simulink library "sm_rollerV_lib_underc_idlerArm_i2u0l3"  (R2026a)
settings: Solver=VariableStepAuto
undefined symbols (not defined in the file): Fixed, P1, P2, P3, P4, P5, Right, Trac, X, Y, Z
libraries: sm_rollerV_lib_underc_elem x11, sm_lib x11, nesl_utility x7, sm_trackV_lib_belt_underc_elem x4, fl_lib x2, sm_trackV_lib_frame_idlerArm_i2u0l3 x1
(part 2 of 2)

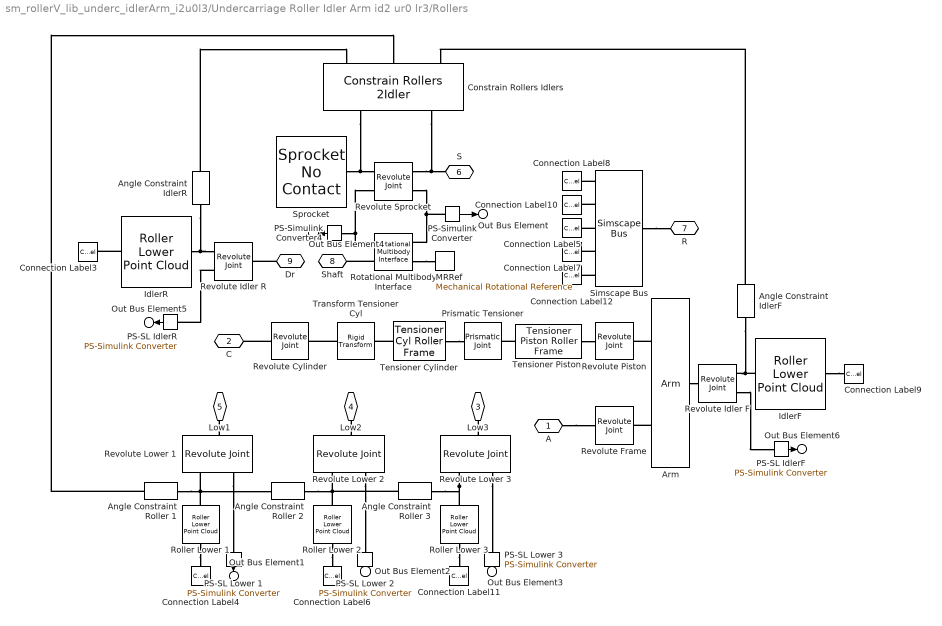
== system sm_rollerV_lib_underc_idlerArm_i2u0l3/Undercarriage Roller Idler Arm id2 ur0 lr3/Rollers ==
  Angle Constraint IdlerF : sm_rollerV_lib_underc_elem/Angle Constraint  SystemSampleTime=-1  VariantActivationTime=update diagram  EmptyChoice=off  PassThrough=off  PassThroughVariantControl=(default)  EmptyChoiceVariantControl=(default)  AllowFlexibleInterface=on  Latency=0  AutoFrameSizeCalculation=off
  Angle Constraint IdlerR : sm_rollerV_lib_underc_elem/Angle Constraint  SystemSampleTime=-1  VariantActivationTime=update diagram  EmptyChoice=off  PassThrough=off  PassThroughVariantControl=(default)  EmptyChoiceVariantControl=(default)  AllowFlexibleInterface=on  Latency=0  AutoFrameSizeCalculation=off
  Angle Constraint Roller 1 : sm_rollerV_lib_underc_elem/Angle Constraint  SystemSampleTime=-1  VariantActivationTime=update diagram  EmptyChoice=off  PassThrough=off  PassThroughVariantControl=(default)  EmptyChoiceVariantControl=(default)  AllowFlexibleInterface=on  Latency=0  AutoFrameSizeCalculation=off
  Angle Constraint Roller 2 : sm_rollerV_lib_underc_elem/Angle Constraint  SystemSampleTime=-1  VariantActivationTime=update diagram  EmptyChoice=off  PassThrough=off  PassThroughVariantControl=(default)  EmptyChoiceVariantControl=(default)  AllowFlexibleInterface=on  Latency=0  AutoFrameSizeCalculation=off
  Angle Constraint Roller 3 : sm_rollerV_lib_underc_elem/Angle Constraint  SystemSampleTime=-1  VariantActivationTime=update diagram  EmptyChoice=off  PassThrough=off  PassThroughVariantControl=(default)  EmptyChoiceVariantControl=(default)  AllowFlexibleInterface=on  Latency=0  AutoFrameSizeCalculation=off
  Arm : sm_trackV_lib_belt_underc_elem/Arm  arm_idlerc=arm_idlerc  arm_tens_x=arm_tens_x  arm_tens_y=arm_tens_y  arm_wid=arm_wid  arm_thk=arm_thk  arm_rho=arm_rho  arm_clr=arm_clr  arm_opc=arm_opc
  Connection Label10 : ConnectionLabel  Label=A
  Connection Label11 : ConnectionLabel  Label=L3
  Connection Label12 : ConnectionLabel  Label=L3
  Connection Label3 : ConnectionLabel  Label=X
  Connection Label4 : ConnectionLabel  Label=L1
  Connection Label5 : ConnectionLabel  Label=L1
  Connection Label6 : ConnectionLabel  Label=L2
  Connection Label7 : ConnectionLabel  Label=L2
  Connection Label8 : ConnectionLabel  Label=X
  Connection Label9 : ConnectionLabel  Label=A
  Constrain Rollers Idlers : sm_rollerV_lib_underc_elem/Constrain Rollers 2Idler  sprk_rolling_rad=sprk_rolling_rad  roller_lower_rolling_rad=roller_lower_rolling_rad  idlerF_rolling_rad=idlerF_rolling_rad  idlerR_rolling_rad=idlerR_rolling_rad
  IdlerF : sm_rollerV_lib_underc_elem/Roller Lower Point Cloud  roller_lower_rad=idlerF_rad  roller_lower_len=idlerF_total_len  roller_lower_rho=idlerF_avg_rho  roller_lower_clr=idlerF_clr  roller_lower_opc=idlerF_opc  roller_lower_contgeo_ptcld=idlerF_contgeo_ptcld  roller_lower_contgeo_rad=idlerF_contgeo_rad  roller_lower_contgeo_clr=idlerF_contgeo_clr  roller_lower_contgeo_opc=idlerF_contgeo_opc  cyl_rad=idlerF_rolling_rad  cyl_len=cyl_len  cyl_clr=idlerF_rollvervis_clr  cyl_opc=idlerF_rollervis_opc  accMn=accMn  accMx=accMx  acc_clr=acc_clr  acc_opc=acc_opc  lext=lext
      settings: LibrarySourceBlock=sm_chain_drive_lib/Pulley_Bot
  IdlerR : sm_rollerV_lib_underc_elem/Roller Lower Point Cloud  roller_lower_rad=idlerR_rad  roller_lower_len=idlerR_total_len  roller_lower_rho=idlerR_avg_rho  roller_lower_clr=idlerR_clr  roller_lower_opc=idlerR_opc  roller_lower_contgeo_ptcld=idlerR_contgeo_ptcld  roller_lower_contgeo_rad=idlerR_contgeo_rad  roller_lower_contgeo_clr=idlerR_contgeo_clr  roller_lower_contgeo_opc=idlerR_contgeo_opc  cyl_rad=idlerR_rolling_rad  cyl_len=cyl_len  cyl_clr=idlerR_rollvervis_clr  cyl_opc=idlerR_rollervis_opc  accMn=accMn  accMx=accMx  acc_clr=acc_clr  acc_opc=acc_opc  lext=lext
      settings: LibrarySourceBlock=sm_chain_drive_lib/Pulley_Bot
  MRRef : fl_lib/Mechanical/Rotational Elements/Mechanical Rotational Reference
  PS-SL IdlerF : nesl_utility/PS-Simulink Converter  PhysicalDomain=network_engine_domain  SubClassName=ps_output  LeftPortType=input  RightPortType=output  PseudoPeriodic=off  Frequencies=[]  VectorFormat=inherit  Unit=inherit  AffineConversion=off
  PS-SL IdlerR : nesl_utility/PS-Simulink Converter  PhysicalDomain=network_engine_domain  SubClassName=ps_output  LeftPortType=input  RightPortType=output  PseudoPeriodic=off  Frequencies=[]  VectorFormat=inherit  Unit=inherit  AffineConversion=off
  PS-SL Lower 1 : nesl_utility/PS-Simulink Converter  PhysicalDomain=network_engine_domain  SubClassName=ps_output  LeftPortType=input  RightPortType=output  PseudoPeriodic=off  Frequencies=[]  VectorFormat=inherit  Unit=inherit  AffineConversion=off
  PS-SL Lower 2 : nesl_utility/PS-Simulink Converter  PhysicalDomain=network_engine_domain  SubClassName=ps_output  LeftPortType=input  RightPortType=output  PseudoPeriodic=off  Frequencies=[]  VectorFormat=inherit  Unit=inherit  AffineConversion=off
  PS-SL Lower 3 : nesl_utility/PS-Simulink Converter  PhysicalDomain=network_engine_domain  SubClassName=ps_output  LeftPortType=input  RightPortType=output  PseudoPeriodic=off  Frequencies=[]  VectorFormat=inherit  Unit=inherit  AffineConversion=off
  PS-Simulink Converter : nesl_utility/PS-Simulink Converter  PhysicalDomain=network_engine_domain  SubClassName=ps_output  LeftPortType=input  RightPortType=output  PseudoPeriodic=off  Frequencies=[]  VectorFormat=inherit  Unit=inherit  AffineConversion=off
  PS-Simulink Converter4 : nesl_utility/PS-Simulink Converter  PhysicalDomain=network_engine_domain  SubClassName=ps_output  LeftPortType=input  RightPortType=output  PseudoPeriodic=off  Frequencies=[]  VectorFormat=inherit  Unit=inherit  AffineConversion=off
  Prismatic Tensioner : sm_lib/Joints/Prismatic Joint  JointMode=Normal  CompositeWrenchDir=FollowerOnBase  CompositeWrenchFrame=BaseFrame  SenseConstraintForce=off  SenseConstraintTorque=off  SenseTotalForce=off  SenseTotalTorque=off  PositionTargetSpecify=on  PositionTargetPriority=High  PositionTargetValue=tensioner_x0  PositionTargetValueUnits=m  VelocityTargetSpecify=off  VelocityTargetPriority=High  VelocityTargetValue=0  VelocityTargetValueUnits=m/s  EquilibriumPosition=tensioner_eqpos  EquilibriumPositionUnits=m  SpringStiffness=tensioner_k  SpringStiffnessUnits=N/m  DampingCoefficient=tensioner_b  DampingCoefficientUnits=N/(m/s)  LowerLimitSpecify=off  LowerLimitBound=-1  LowerLimitBoundUnits=m  LowerLimitStiffness=1e6  LowerLimitStiffnessUnits=N/m  LowerLimitDamping=1e3  LowerLimitDampingUnits=N/(m/s)  LowerLimitTransitionRegionWidth=1e-4  LowerLimitTransitionRegionWidthUnits=m  UpperLimitSpecify=off  UpperLimitBound=1  UpperLimitBoundUnits=m  UpperLimitStiffness=1e6  UpperLimitStiffnessUnits=N/m  UpperLimitDamping=1e3  UpperLimitDampingUnits=N/(m/s)  UpperLimitTransitionRegionWidth=1e-4  UpperLimitTransitionRegionWidthUnits=m  TorqueActuationMode=NoTorque  MotionActuationMode=ComputedMotion  SensePosition=off  SenseVelocity=off  SenseAcceleration=off  SenseTorqueForce=off  SenseLowerLimitTorqueForce=off  SenseUpperLimitTorqueForce=off
  Revolute Cylinder : sm_lib/Joints/Revolute Joint  JointMode=Normal  CompositeWrenchDir=FollowerOnBase  CompositeWrenchFrame=BaseFrame  SenseConstraintForce=off  SenseConstraintTorque=off  SenseTotalForce=off  SenseTotalTorque=off  PositionTargetSpecify=on  PositionTargetPriority=Low  PositionTargetValue=0  PositionTargetValueUnits=deg  VelocityTargetSpecify=off  VelocityTargetPriority=High  VelocityTargetValue=0  VelocityTargetValueUnits=deg/s  EquilibriumPosition=0  EquilibriumPositionUnits=deg  SpringStiffness=0  SpringStiffnessUnits=N*m/deg  DampingCoefficient=0  DampingCoefficientUnits=N*m/(deg/s)  LowerLimitSpecify=off  LowerLimitBound=-90  LowerLimitBoundUnits=deg  LowerLimitStiffness=1e4  LowerLimitStiffnessUnits=N*m/deg  LowerLimitDamping=10  LowerLimitDampingUnits=N*m/(deg/s)  LowerLimitTransitionRegionWidth=0.1  LowerLimitTransitionRegionWidthUnits=deg  UpperLimitSpecify=off  UpperLimitBound=90  UpperLimitBoundUnits=deg  UpperLimitStiffness=1e4  UpperLimitStiffnessUnits=N*m/deg  UpperLimitDamping=10  UpperLimitDampingUnits=N*m/(deg/s)  UpperLimitTransitionRegionWidth=0.1  UpperLimitTransitionRegionWidthUnits=deg  TorqueActuationMode=NoTorque  MotionActuationMode=ComputedMotion  SensePosition=off  SenseVelocity=off  SenseAcceleration=off  SenseTorqueForce=off  SenseLowerLimitTorqueForce=off  SenseUpperLimitTorqueForce=off
  Revolute Frame : sm_lib/Joints/Revolute Joint  JointMode=Normal  CompositeWrenchDir=FollowerOnBase  CompositeWrenchFrame=BaseFrame  SenseConstraintForce=off  SenseConstraintTorque=off  SenseTotalForce=off  SenseTotalTorque=off  PositionTargetSpecify=off  PositionTargetPriority=Low  PositionTargetValue=0  PositionTargetValueUnits=deg  VelocityTargetSpecify=off  VelocityTargetPriority=High  VelocityTargetValue=0  VelocityTargetValueUnits=deg/s  EquilibriumPosition=0  EquilibriumPositionUnits=rad  SpringStiffness=0  SpringStiffnessUnits=N*m/rad  DampingCoefficient=0  DampingCoefficientUnits=N*m/(rad/s)  LowerLimitSpecify=off  LowerLimitBound=-90  LowerLimitBoundUnits=deg  LowerLimitStiffness=1e4  LowerLimitStiffnessUnits=N*m/deg  LowerLimitDamping=10  LowerLimitDampingUnits=N*m/(deg/s)  LowerLimitTransitionRegionWidth=0.1  LowerLimitTransitionRegionWidthUnits=deg  UpperLimitSpecify=off  UpperLimitBound=90  UpperLimitBoundUnits=deg  UpperLimitStiffness=1e4  UpperLimitStiffnessUnits=N*m/deg  UpperLimitDamping=10  UpperLimitDampingUnits=N*m/(deg/s)  UpperLimitTransitionRegionWidth=0.1  UpperLimitTransitionRegionWidthUnits=deg  TorqueActuationMode=NoTorque  MotionActuationMode=ComputedMotion  SensePosition=off  SenseVelocity=off  SenseAcceleration=off  SenseTorqueForce=off  SenseLowerLimitTorqueForce=off  SenseUpperLimitTorqueForce=off
  Revolute Idler F : sm_lib/Joints/Revolute Joint  JointMode=Normal  CompositeWrenchDir=FollowerOnBase  CompositeWrenchFrame=BaseFrame  SenseConstraintForce=off  SenseConstraintTorque=off  SenseTotalForce=off  SenseTotalTorque=off  PositionTargetSpecify=off  PositionTargetPriority=Low  PositionTargetValue=0  PositionTargetValueUnits=deg  VelocityTargetSpecify=off  VelocityTargetPriority=High  VelocityTargetValue=0  VelocityTargetValueUnits=deg/s  EquilibriumPosition=0  EquilibriumPositionUnits=rad  SpringStiffness=0  SpringStiffnessUnits=N*m/rad  DampingCoefficient=0  DampingCoefficientUnits=N*m/(rad/s)  LowerLimitSpecify=off  LowerLimitBound=-90  LowerLimitBoundUnits=deg  LowerLimitStiffness=1e4  LowerLimitStiffnessUnits=N*m/deg  LowerLimitDamping=10  LowerLimitDampingUnits=N*m/(deg/s)  LowerLimitTransitionRegionWidth=0.1  LowerLimitTransitionRegionWidthUnits=deg  UpperLimitSpecify=off  UpperLimitBound=90  UpperLimitBoundUnits=deg  UpperLimitStiffness=1e4  UpperLimitStiffnessUnits=N*m/deg  UpperLimitDamping=10  UpperLimitDampingUnits=N*m/(deg/s)  UpperLimitTransitionRegionWidth=0.1  UpperLimitTransitionRegionWidthUnits=deg  TorqueActuationMode=NoTorque  MotionActuationMode=ComputedMotion  SensePosition=off  SenseVelocity=off  SenseAcceleration=off  SenseTorqueForce=on  SenseLowerLimitTorqueForce=off  SenseUpperLimitTorqueForce=off
  Revolute Idler R : sm_lib/Joints/Revolute Joint  JointMode=Normal  CompositeWrenchDir=FollowerOnBase  CompositeWrenchFrame=BaseFrame  SenseConstraintForce=off  SenseConstraintTorque=off  SenseTotalForce=off  SenseTotalTorque=off  PositionTargetSpecify=off  PositionTargetPriority=Low  PositionTargetValue=0  PositionTargetValueUnits=deg  VelocityTargetSpecify=off  VelocityTargetPriority=High  VelocityTargetValue=0  VelocityTargetValueUnits=deg/s  EquilibriumPosition=0  EquilibriumPositionUnits=rad  SpringStiffness=0  SpringStiffnessUnits=N*m/rad  DampingCoefficient=0  DampingCoefficientUnits=N*m/(rad/s)  LowerLimitSpecify=off  LowerLimitBound=-90  LowerLimitBoundUnits=deg  LowerLimitStiffness=1e4  LowerLimitStiffnessUnits=N*m/deg  LowerLimitDamping=10  LowerLimitDampingUnits=N*m/(deg/s)  LowerLimitTransitionRegionWidth=0.1  LowerLimitTransitionRegionWidthUnits=deg  UpperLimitSpecify=off  UpperLimitBound=90  UpperLimitBoundUnits=deg  UpperLimitStiffness=1e4  UpperLimitStiffnessUnits=N*m/deg  UpperLimitDamping=10  UpperLimitDampingUnits=N*m/(deg/s)  UpperLimitTransitionRegionWidth=0.1  UpperLimitTransitionRegionWidthUnits=deg  TorqueActuationMode=NoTorque  MotionActuationMode=ComputedMotion  SensePosition=off  SenseVelocity=off  SenseAcceleration=off  SenseTorqueForce=on  SenseLowerLimitTorqueForce=off  SenseUpperLimitTorqueForce=off
  Revolute Lower 1 : sm_lib/Joints/Revolute Joint  JointMode=Normal  CompositeWrenchDir=FollowerOnBase  CompositeWrenchFrame=BaseFrame  SenseConstraintForce=off  SenseConstraintTorque=off  SenseTotalForce=off  SenseTotalTorque=off  PositionTargetSpecify=off  PositionTargetPriority=Low  PositionTargetValue=0  PositionTargetValueUnits=deg  VelocityTargetSpecify=off  VelocityTargetPriority=High  VelocityTargetValue=0  VelocityTargetValueUnits=deg/s  EquilibriumPosition=0  EquilibriumPositionUnits=rad  SpringStiffness=0  SpringStiffnessUnits=N*m/rad  DampingCoefficient=0  DampingCoefficientUnits=N*m/(rad/s)  LowerLimitSpecify=off  LowerLimitBound=-90  LowerLimitBoundUnits=deg  LowerLimitStiffness=1e4  LowerLimitStiffnessUnits=N*m/deg  LowerLimitDamping=10  LowerLimitDampingUnits=N*m/(deg/s)  LowerLimitTransitionRegionWidth=0.1  LowerLimitTransitionRegionWidthUnits=deg  UpperLimitSpecify=off  UpperLimitBound=90  UpperLimitBoundUnits=deg  UpperLimitStiffness=1e4  UpperLimitStiffnessUnits=N*m/deg  UpperLimitDamping=10  UpperLimitDampingUnits=N*m/(deg/s)  UpperLimitTransitionRegionWidth=0.1  UpperLimitTransitionRegionWidthUnits=deg  TorqueActuationMode=NoTorque  MotionActuationMode=ComputedMotion  SensePosition=off  SenseVelocity=off  SenseAcceleration=off  SenseTorqueForce=on  SenseLowerLimitTorqueForce=off  SenseUpperLimitTorqueForce=off
  Revolute Lower 2 : sm_lib/Joints/Revolute Joint  JointMode=Normal  CompositeWrenchDir=FollowerOnBase  CompositeWrenchFrame=BaseFrame  SenseConstraintForce=off  SenseConstraintTorque=off  SenseTotalForce=off  SenseTotalTorque=off  PositionTargetSpecify=off  PositionTargetPriority=Low  PositionTargetValue=0  PositionTargetValueUnits=deg  VelocityTargetSpecify=off  VelocityTargetPriority=High  VelocityTargetValue=0  VelocityTargetValueUnits=deg/s  EquilibriumPosition=0  EquilibriumPositionUnits=rad  SpringStiffness=0  SpringStiffnessUnits=N*m/rad  DampingCoefficient=0  DampingCoefficientUnits=N*m/(rad/s)  LowerLimitSpecify=off  LowerLimitBound=-90  LowerLimitBoundUnits=deg  LowerLimitStiffness=1e4  LowerLimitStiffnessUnits=N*m/deg  LowerLimitDamping=10  LowerLimitDampingUnits=N*m/(deg/s)  LowerLimitTransitionRegionWidth=0.1  LowerLimitTransitionRegionWidthUnits=deg  UpperLimitSpecify=off  UpperLimitBound=90  UpperLimitBoundUnits=deg  UpperLimitStiffness=1e4  UpperLimitStiffnessUnits=N*m/deg  UpperLimitDamping=10  UpperLimitDampingUnits=N*m/(deg/s)  UpperLimitTransitionRegionWidth=0.1  UpperLimitTransitionRegionWidthUnits=deg  TorqueActuationMode=NoTorque  MotionActuationMode=ComputedMotion  SensePosition=off  SenseVelocity=off  SenseAcceleration=off  SenseTorqueForce=on  SenseLowerLimitTorqueForce=off  SenseUpperLimitTorqueForce=off
  Revolute Lower 3 : sm_lib/Joints/Revolute Joint  JointMode=Normal  CompositeWrenchDir=FollowerOnBase  CompositeWrenchFrame=BaseFrame  SenseConstraintForce=off  SenseConstraintTorque=off  SenseTotalForce=off  SenseTotalTorque=off  PositionTargetSpecify=off  PositionTargetPriority=Low  PositionTargetValue=0  PositionTargetValueUnits=deg  VelocityTargetSpecify=off  VelocityTargetPriority=High  VelocityTargetValue=0  VelocityTargetValueUnits=deg/s  EquilibriumPosition=0  EquilibriumPositionUnits=rad  SpringStiffness=0  SpringStiffnessUnits=N*m/rad  DampingCoefficient=0  DampingCoefficientUnits=N*m/(rad/s)  LowerLimitSpecify=off  LowerLimitBound=-90  LowerLimitBoundUnits=deg  LowerLimitStiffness=1e4  LowerLimitStiffnessUnits=N*m/deg  LowerLimitDamping=10  LowerLimitDampingUnits=N*m/(deg/s)  LowerLimitTransitionRegionWidth=0.1  LowerLimitTransitionRegionWidthUnits=deg  UpperLimitSpecify=off  UpperLimitBound=90  UpperLimitBoundUnits=deg  UpperLimitStiffness=1e4  UpperLimitStiffnessUnits=N*m/deg  UpperLimitDamping=10  UpperLimitDampingUnits=N*m/(deg/s)  UpperLimitTransitionRegionWidth=0.1  UpperLimitTransitionRegionWidthUnits=deg  TorqueActuationMode=NoTorque  MotionActuationMode=ComputedMotion  SensePosition=off  SenseVelocity=off  SenseAcceleration=off  SenseTorqueForce=on  SenseLowerLimitTorqueForce=off  SenseUpperLimitTorqueForce=off
  Revolute Piston : sm_lib/Joints/Revolute Joint  JointMode=Normal  CompositeWrenchDir=FollowerOnBase  CompositeWrenchFrame=BaseFrame  SenseConstraintForce=off  SenseConstraintTorque=off  SenseTotalForce=off  SenseTotalTorque=off  PositionTargetSpecify=off  PositionTargetPriority=Low  PositionTargetValue=0  PositionTargetValueUnits=deg  VelocityTargetSpecify=off  VelocityTargetPriority=High  VelocityTargetValue=0  VelocityTargetValueUnits=deg/s  EquilibriumPosition=0  EquilibriumPositionUnits=rad  SpringStiffness=0  SpringStiffnessUnits=N*m/rad  DampingCoefficient=0  DampingCoefficientUnits=N*m/(rad/s)  LowerLimitSpecify=off  LowerLimitBound=-90  LowerLimitBoundUnits=deg  LowerLimitStiffness=1e4  LowerLimitStiffnessUnits=N*m/deg  LowerLimitDamping=10  LowerLimitDampingUnits=N*m/(deg/s)  LowerLimitTransitionRegionWidth=0.1  LowerLimitTransitionRegionWidthUnits=deg  UpperLimitSpecify=off  UpperLimitBound=90  UpperLimitBoundUnits=deg  UpperLimitStiffness=1e4  UpperLimitStiffnessUnits=N*m/deg  UpperLimitDamping=10  UpperLimitDampingUnits=N*m/(deg/s)  UpperLimitTransitionRegionWidth=0.1  UpperLimitTransitionRegionWidthUnits=deg  TorqueActuationMode=NoTorque  MotionActuationMode=ComputedMotion  SensePosition=off  SenseVelocity=off  SenseAcceleration=off  SenseTorqueForce=off  SenseLowerLimitTorqueForce=off  SenseUpperLimitTorqueForce=off
  Revolute Sprocket : sm_lib/Joints/Revolute Joint  JointMode=Normal  CompositeWrenchDir=FollowerOnBase  CompositeWrenchFrame=BaseFrame  SenseConstraintForce=off  SenseConstraintTorque=off  SenseTotalForce=off  SenseTotalTorque=off  PositionTargetSpecify=off  PositionTargetPriority=Low  PositionTargetValue=0  PositionTargetValueUnits=deg  VelocityTargetSpecify=off  VelocityTargetPriority=High  VelocityTargetValue=0  VelocityTargetValueUnits=deg/s  EquilibriumPosition=0  EquilibriumPositionUnits=rad  SpringStiffness=0  SpringStiffnessUnits=N*m/rad  DampingCoefficient=0  DampingCoefficientUnits=N*m/(rad/s)  LowerLimitSpecify=off  LowerLimitBound=-90  LowerLimitBoundUnits=deg  LowerLimitStiffness=1e4  LowerLimitStiffnessUnits=N*m/deg  LowerLimitDamping=10  LowerLimitDampingUnits=N*m/(deg/s)  LowerLimitTransitionRegionWidth=0.1  LowerLimitTransitionRegionWidthUnits=deg  UpperLimitSpecify=off  UpperLimitBound=90  UpperLimitBoundUnits=deg  UpperLimitStiffness=1e4  UpperLimitStiffnessUnits=N*m/deg  UpperLimitDamping=10  UpperLimitDampingUnits=N*m/(deg/s)  UpperLimitTransitionRegionWidth=0.1  UpperLimitTransitionRegionWidthUnits=deg  TorqueActuationMode=InputTorque  MotionActuationMode=ComputedMotion  SensePosition=off  SenseVelocity=on  SenseAcceleration=off  SenseTorqueForce=off  SenseLowerLimitTorqueForce=off  SenseUpperLimitTorqueForce=off
  Roller Lower 1 : sm_rollerV_lib_underc_elem/Roller Lower Point Cloud  roller_lower_rad=roller_lower_rad  roller_lower_len=roller_lower_len  roller_lower_rho=roller_lower_rho  roller_lower_clr=roller_lower_clr  roller_lower_opc=roller_lower_opc  roller_lower_contgeo_ptcld=roller_lower_contgeo_ptcld  roller_lower_contgeo_rad=roller_lower_contgeo_rad  roller_lower_contgeo_clr=roller_lower_contgeo_clr  roller_lower_contgeo_opc=roller_lower_contgeo_opc  cyl_rad=roller_lower_rolling_rad  cyl_len=cyl_len  cyl_clr=roller_lower_cyl_clr  cyl_opc=roller_lower_cyl_opc  accMn=accMn  accMx=accMx  acc_clr=acc_clr  acc_opc=acc_opc  lext=lext
      settings: LibrarySourceBlock=sm_chain_drive_lib/Pulley_Bot
  Roller Lower 2 : sm_rollerV_lib_underc_elem/Roller Lower Point Cloud  roller_lower_rad=roller_lower_rad  roller_lower_len=roller_lower_len  roller_lower_rho=roller_lower_rho  roller_lower_clr=roller_lower_clr  roller_lower_opc=roller_lower_opc  roller_lower_contgeo_ptcld=roller_lower_contgeo_ptcld  roller_lower_contgeo_rad=roller_lower_contgeo_rad  roller_lower_contgeo_clr=roller_lower_contgeo_clr  roller_lower_contgeo_opc=roller_lower_contgeo_opc  cyl_rad=roller_lower_rolling_rad  cyl_len=cyl_len  cyl_clr=roller_lower_cyl_clr  cyl_opc=roller_lower_cyl_opc  accMn=accMn  accMx=accMx  acc_clr=acc_clr  acc_opc=acc_opc  lext=lext
      settings: LibrarySourceBlock=sm_chain_drive_lib/Pulley_Bot
  Roller Lower 3 : sm_rollerV_lib_underc_elem/Roller Lower Point Cloud  roller_lower_rad=roller_lower_rad  roller_lower_len=roller_lower_len  roller_lower_rho=roller_lower_rho  roller_lower_clr=roller_lower_clr  roller_lower_opc=roller_lower_opc  roller_lower_contgeo_ptcld=roller_lower_contgeo_ptcld  roller_lower_contgeo_rad=roller_lower_contgeo_rad  roller_lower_contgeo_clr=roller_lower_contgeo_clr  roller_lower_contgeo_opc=roller_lower_contgeo_opc  cyl_rad=roller_lower_rolling_rad  cyl_len=cyl_len  cyl_clr=roller_lower_cyl_clr  cyl_opc=roller_lower_cyl_opc  accMn=accMn  accMx=accMx  acc_clr=acc_clr  acc_opc=acc_opc  lext=lext
      settings: LibrarySourceBlock=sm_chain_drive_lib/Pulley_Bot
  Rotational Multibody Interface : fl_lib/Mechanical/Multibody Interfaces/Rotational Multibody Interface
  Simscape Bus : SimscapeBus  HierarchyStrings=P1;P2;P3;P4;P5
  Sprocket : sm_trackV_lib_belt_underc_elem/Sprocket No Contact  sprk_wid_roll=sprk_wid_roll  sprk_rad_roll=sprk_rad_roll  sprk_opc=sprk_opc  sprk_clr=sprk_clr  sprk_rad_pitch=sprk_rad_pitch  sprk_spoke_rad=sprk_spoke_rad  sprk_spoke_len=sprk_spoke_len  sprk_spoke_num=sprk_spoke_num  sprk_spoke_clr=sprk_clr  sprk_spoke_opc=sprk_opc  rim_spoke_xc=sprk_rim_spoke_xc  rim_thk=sprk_rim_thk  rim_ir=sprk_rim_ir
  Tensioner Cylinder : sm_trackV_lib_belt_underc_elem/Tensioner Cyl Roller Frame  cyl_rad=tensioner_cyl_rad  cyl_len=tensioner_cyl_len  cyl_rho=tensioner_cyl_rho  cyl_clr=tensioner_cyl_clr  cyl_opc=tensioner_cyl_opc
  Tensioner Piston : sm_trackV_lib_belt_underc_elem/Tensioner Piston Roller Frame  pist_rad=tensioner_pist_rad  pist_len=pist_len  pist_rho=tensioner_pist_rho  pist_clr=tensioner_pist_clr  pist_opc=tensioner_pist_opc  br_height=tensioner_br_height  br_length=brk_len  br_width=tensioner_br_width  br_rho=tensioner_br_rho  br_thk=brk_thk  br_clr=tensioner_br_clr  br_opc=tensioner_br_opc
  Transform Tensioner Cyl : sm_lib/Frames and Transforms/Rigid Transform  RotationMethod=AlignedAxes  FollAlignAxisA=+Z  BaseAlignAxisA=+X  FollAlignAxisB=+X  BaseAlignAxisB=+Y  RotationStandardAxis=+Y  RotationAngle=90  RotationAngleUnits=deg  RotationArbitraryAxis=[0 0 1]  RotationSequenceAxes=FollowerAxes  RotationSequence=XYX  RotationSequenceAngles=[0 0 0]  RotationSequenceAnglesUnits=deg  RotationMatrix=[1 0 0; 0 1 0; 0 0 1]  Quaternion=[1 0 0 0]  TranslationMethod=None  TranslationCartesianOffset=[0 0 0]  TranslationCartesianOffsetUnits=m  TranslationStandardAxis=+Z  TranslationStandardOffset=0  TranslationStandardOffsetUnits=m  TranslationROffset=0  TranslationROffsetUnits=m  TranslationThetaOffset=0  TranslationThetaOffsetUnits=deg  TranslationZOffset=0  TranslationZOffsetUnits=m
  A : PMIOPort  Side=Left
  C : PMIOPort  Port=2  Side=Left
  Low3 : PMIOPort  Port=3  Side=Left
  Low2 : PMIOPort  Port=4  Side=Left
  Low1 : PMIOPort  Port=5  Side=Left
  S : PMIOPort  Port=6  Side=Left
  R : PMIOPort  Port=7  Side=Right
  Shaft : PMIOPort  Port=8  Side=Right
  Dr : PMIOPort  Port=9  Side=Left
  Out Bus Element : Outport  PortName=m  Element=tSprk
  Out Bus Element1 : Outport  PortName=m  Element=RL1
  Out Bus Element2 : Outport  PortName=m  Element=RL2
  Out Bus Element3 : Outport  PortName=m  Element=RL3
  Out Bus Element4 : Outport  PortName=m  Element=wSprk
  Out Bus Element5 : Outport  PortName=m  Element=XIdlerR
  Out Bus Element6 : Outport  PortName=m  Element=XIdlerF
  wires:
  PS-Simulink Converter/1 -> Out Bus Element/1
  PS-SL Lower 1/1 -> Out Bus Element1/1
  PS-SL Lower 2/1 -> Out Bus Element2/1
  PS-SL Lower 3/1 -> Out Bus Element3/1
  PS-Simulink Converter4/1 -> Out Bus Element4/1
  PS-SL IdlerR/1 -> Out Bus Element5/1
  PS-SL IdlerF/1 -> Out Bus Element6/1
  connections:
  A/RConn1 -- Revolute Frame/LConn1
  Arm/LConn2 -- Revolute Frame/RConn1
  Tensioner Piston/RConn1 -- Revolute Piston/LConn1
  Arm/LConn1 -- Revolute Piston/RConn1
  Arm/RConn1 -- Revolute Idler F/LConn1
  IdlerF/RConn1 -- Connection Label9/LConn1
  Roller Lower 2/RConn1 -- Connection Label6/LConn1
  Revolute Sprocket/LConn1 -- Constrain Rollers Idlers/LConn2 -- S/RConn1
  Simscape Bus/RConn1 -- R/RConn1
  IdlerF/LConn1 -- Angle Constraint IdlerF/RConn1 -- Revolute Idler F/RConn1
  Revolute Sprocket/RConn1 -- Constrain Rollers Idlers/LConn1 -- Sprocket/RConn1
  Tensioner Cylinder/RConn1 -- Prismatic Tensioner/LConn1
  Revolute Lower 2/LConn1 -- Low2/RConn1
  Roller Lower 1/RConn1 -- Connection Label4/LConn1
  Revolute Lower 1/LConn1 -- Low1/RConn1
  Simscape Bus/LConn1 -- Connection Label8/LConn1
  Tensioner Cylinder/LConn1 -- Transform Tensioner Cyl/RConn1
  Tensioner Piston/LConn1 -- Prismatic Tensioner/RConn1
  Angle Constraint Roller 2/RConn1 -- Roller Lower 2/LConn1 -- Angle Constraint Roller 3/LConn1 -- Revolute Lower 2/RConn1
  Angle Constraint Roller 1/RConn1 -- Roller Lower 1/LConn1 -- Angle Constraint Roller 2/LConn1 -- Revolute Lower 1/RConn1
  Revolute Sprocket/LConn2 -- Rotational Multibody Interface/LConn1 -- PS-Simulink Converter/LConn1
  Rotational Multibody Interface/RConn1 -- PS-Simulink Converter4/LConn1 -- Revolute Sprocket/RConn2
  Rotational Multibody Interface/RConn2 -- Shaft/RConn1
  Rotational Multibody Interface/LConn2 -- MRRef/LConn1
  IdlerR/LConn1 -- Angle Constraint IdlerR/RConn1 -- Revolute Idler R/RConn1
  Dr/RConn1 -- Revolute Idler R/LConn1
  Transform Tensioner Cyl/LConn1 -- Revolute Cylinder/RConn1
  Revolute Cylinder/LConn1 -- C/RConn1
  Simscape Bus/LConn2 -- Connection Label10/LConn1
  IdlerR/RConn1 -- Connection Label3/LConn1
  Simscape Bus/LConn3 -- Connection Label5/LConn1
  Simscape Bus/LConn4 -- Connection Label7/LConn1
  Revolute Lower 3/RConn1 -- Roller Lower 3/LConn1 -- Angle Constraint Roller 3/RConn1
  Revolute Lower 3/LConn1 -- Low3/RConn1
  Roller Lower 3/RConn1 -- Connection Label11/LConn1
  Simscape Bus/LConn5 -- Connection Label12/LConn1
  Angle Constraint Roller 1/LConn1 -- Constrain Rollers Idlers/RConn2
  Angle Constraint IdlerF/LConn1 -- Constrain Rollers Idlers/RConn3
  Angle Constraint IdlerR/LConn1 -- Constrain Rollers Idlers/RConn1
  Revolute Lower 1/RConn2 -- PS-SL Lower 1/LConn1
  Revolute Lower 2/RConn2 -- PS-SL Lower 2/LConn1
  Revolute Lower 3/RConn2 -- PS-SL Lower 3/LConn1
  Revolute Idler R/RConn2 -- PS-SL IdlerR/LConn1
  Revolute Idler F/RConn2 -- PS-SL IdlerF/LConn1
